simulink model "RBCM_Model"  (R2024b)
settings: Solver=FixedStepAuto  StartTime=0.0  StopTime=10.0  RelTol=1e-3
PreLoadFcn:
  | % NXP_MBDT_S32K3 callback: DO NOT REMOVE
  | mbd_s32k3.common.nxp.model_callbacks.preLoadFcn();
PostLoadFcn:
  | % NXP_MBDT_S32K3 callback: DO NOT REMOVE
  | mbd_s32k3.common.nxp.model_callbacks.postLoadFcn();
InitFcn:
  | % NXP_MBDT_S32K3 callback: DO NOT REMOVE
  | mbd_s32k3.common.nxp.model_callbacks.initFcn();
undefined symbols (not defined in the file or in its folder): AccuFanPwr_hHsd3ch2, BspdPwr_lHsd1ch2, BuzzerPwr_lHsd3ch3, DevicePwr_12v_lHsd1ch1, DevicePwr_hHsd1ch2, DrsPwr_8v_lHsd3ch1, hHsd_Diagnose_AdcBuffer, ILPwr_hHsd1ch1, lHsd_Diagnose_AdcBuffer, LoggerPwr_lHsd1ch3, PumpFan1_hHsd4ch1, PumpFan2_hHsd4ch2, PumpPwr_hHsd3ch1, RGBLED0state, TaillightPwr_lHsd3ch4, TempSensorPwr_lHsd1ch4
libraries: mbd_s32k3_io_library x127, simulink x48, canmsglib x8, mbd_s32k3_communication_library x7, mbd_s32k3_isr_library x6, mbd_s32k3_cdd_library x3, mbd_s32k3_utility_library x1
(part 2 of 10)

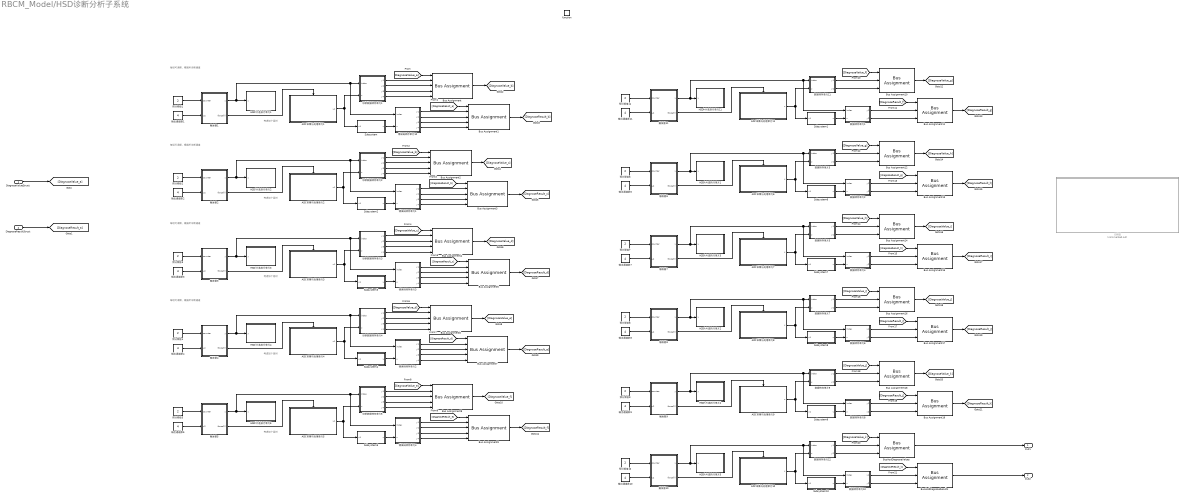
== system RBCM_Model/HSD诊断分析子系统 ==
  note: 考虑加个延时
  note: 每组可调频，根据所诊断通道
  note: 考虑加个延时
  note: 每组可调频，根据所诊断通道
  note: 考虑加个延时
  note: 每组可调频，根据所诊断通道
  note: 考虑加个延时
  note: 每组可调频，根据所诊断通道
  note: 考虑加个延时
  DiagnoseValueStruct : Inport  OutDataTypeStr=Bus: Bus_Hsd_Diagnose_Values
  DiagnoseResultStruct : Inport  Port=2  OutDataTypeStr=Bus: Bus_Hsd_Diagnose_Results
  function : TriggerPort  TriggerType=function-call  VariantControl=Variant
  ADC采集与处理单元1 : Subsystem
  ADC采集与处理单元10 : Subsystem
  ADC采集与处理单元11 : Subsystem
  ADC采集与处理单元2 : Subsystem
  ADC采集与处理单元3 : Subsystem
  ADC采集与处理单元4 : Subsystem
  ADC采集与处理单元5 : Subsystem
  ADC采集与处理单元6 : Subsystem
  ADC采集与处理单元7 : Subsystem
  ADC采集与处理单元8 : Subsystem
  ADC采集与处理单元9 : Subsystem
  Bus Assignment{,1..9} (10 alike) : BusAssignment  AssignedSignals=DevicePwr_12v_lHsd1ch1,BspdPwr_lHsd1ch2,LoggerPwr_lHsd1ch3,TempSensorPwr_lHsd1ch4
  Bus Assignment{10..19} (10 alike) : BusAssignment  AssignedSignals=ILPwr_hHsd1ch1,DevicePwr_hHsd1ch2
  BusHsdDiagnoseResults : BusAssignment  AssignedSignals=ILPwr_hHsd1ch1,DevicePwr_hHsd1ch2
  BusHsdDiagnoseValues : BusAssignment  AssignedSignals=ILPwr_hHsd1ch1,DevicePwr_hHsd1ch2
  HSDh片选执行单元1 : Subsystem
  HSDh片选执行单元11 : Subsystem
  HSDh片选执行单元2 : Subsystem
  HSDh片选执行单元3 : Subsystem
  HSDh片选执行单元4 : Subsystem
  HSDh片选执行单元5 : Subsystem
  HSDl片选执行单元1 : Subsystem
  HSDl片选执行单元2 : Subsystem
  HSDl片选执行单元3 : Subsystem
  HSDl片选执行单元4 : Subsystem
  HSDl片选执行单元5 : Subsystem
  Subsystem : Subsystem
  Subsystem1 : Subsystem
  Subsystem10 : Subsystem
  Subsystem2 : Subsystem
  Subsystem3 : Subsystem
  Subsystem4 : Subsystem
  Subsystem5 : Subsystem
  Subsystem6 : Subsystem
  Subsystem7 : Subsystem
  Subsystem8 : Subsystem
  Subsystem9 : Subsystem
  数据转存单元1 : MATLAB Function  TreatAsAtomicUnit=on
  数据转存单元10 : MATLAB Function  TreatAsAtomicUnit=on
  数据转存单元11 : MATLAB Function  TreatAsAtomicUnit=on
  数据转存单元12 : MATLAB Function  TreatAsAtomicUnit=on
  数据转存单元2 : MATLAB Function  TreatAsAtomicUnit=on
  数据转存单元3 : MATLAB Function  TreatAsAtomicUnit=on
  数据转存单元4 : MATLAB Function  TreatAsAtomicUnit=on
  数据转存单元5 : MATLAB Function  TreatAsAtomicUnit=on
  数据转存单元6 : MATLAB Function  TreatAsAtomicUnit=on
  数据转存单元7 : MATLAB Function  TreatAsAtomicUnit=on
  数据转存单元8 : MATLAB Function  TreatAsAtomicUnit=on
  数据转存单元9 : MATLAB Function  TreatAsAtomicUnit=on
  旧模型 : Subsystem  Commented=on
  触发器1 : MATLAB Function  TreatAsAtomicUnit=on
  触发器10 : MATLAB Function  TreatAsAtomicUnit=on
  触发器11 : MATLAB Function  TreatAsAtomicUnit=on
  触发器2 : MATLAB Function  TreatAsAtomicUnit=on
  触发器3 : MATLAB Function  TreatAsAtomicUnit=on
  触发器4 : MATLAB Function  TreatAsAtomicUnit=on
  触发器5 : MATLAB Function  TreatAsAtomicUnit=on
  触发器6 : MATLAB Function  TreatAsAtomicUnit=on
  触发器7 : MATLAB Function  TreatAsAtomicUnit=on
  触发器8 : MATLAB Function  TreatAsAtomicUnit=on
  触发器9 : MATLAB Function  TreatAsAtomicUnit=on
  诊断数据转存单元1 : MATLAB Function  TreatAsAtomicUnit=on
  诊断数据转存单元2 : MATLAB Function  TreatAsAtomicUnit=on
  诊断数据转存单元3 : MATLAB Function  TreatAsAtomicUnit=on
  诊断数据转存单元4 : MATLAB Function  TreatAsAtomicUnit=on
  诊断数据转存单元5 : MATLAB Function  TreatAsAtomicUnit=on
  输出通道数{1..11} (11 alike) : Constant  Value=4  OutDataTypeStr=uint8
  错误码转存单元1 : MATLAB Function  TreatAsAtomicUnit=on
  错误码转存单元10 : MATLAB Function  TreatAsAtomicUnit=on
  错误码转存单元2 : MATLAB Function  TreatAsAtomicUnit=on
  错误码转存单元3 : MATLAB Function  TreatAsAtomicUnit=on
  错误码转存单元4 : MATLAB Function  TreatAsAtomicUnit=on
  预分频值{1..11} (11 alike) : Constant  Value=2  OutDataTypeStr=uint8
  Out1 : Outport
  Out2 : Outport  Port=2
  wires:
  触发器1/2(fcncall()) -> ADC采集与处理单元1/Trigger
  触发器11/2(fcncall()) -> ADC采集与处理单元11/Trigger
  触发器11/1(y) -> HSDh片选执行单元11/1(y), 数据转存单元1/1(index), 数据转存单元11/1(index)
  触发器1/1(y) -> HSDl片选执行单元1/1(y), 错误码转存单元10/1(index), 诊断数据转存单元1/1(index)
  预分频值1/1 -> 触发器1/1(counter)
  预分频值11/1 -> 触发器11/1(counter)
  输出通道数11/1 -> 触发器11/2(u2)
  输出通道数1/1 -> 触发器1/2(u2)
  数据转存单元11/2(y2) -> Bus Assignment10/3
  数据转存单元11/1(y1) -> Bus Assignment10/2
  ADC采集与处理单元1/1(u1) -> 诊断数据转存单元1/2(u), Subsystem/1(u1)
  ADC采集与处理单元11/1(u) -> Subsystem1/1(u1), 数据转存单元11/2(u)
  Subsystem/1(u) -> 错误码转存单元10/2(u)
  Subsystem1/1(u) -> 数据转存单元1/2(u)
  数据转存单元1/1(y1) -> Bus Assignment11/2
  数据转存单元1/2(y2) -> Bus Assignment11/3
  错误码转存单元10/1(y1) -> Bus Assignment1/2
  诊断数据转存单元1/1(y1) -> Bus Assignment/2
  诊断数据转存单元1/2(y2) -> Bus Assignment/3
  诊断数据转存单元1/3(y3) -> Bus Assignment/4
  诊断数据转存单元1/4(y4) -> Bus Assignment/5
  Subsystem2/1(u) -> 错误码转存单元1/2(u)
  输出通道数2/1 -> 触发器2/2(u2)
  预分频值2/1 -> 触发器2/1(counter)
  触发器2/1(y) -> 诊断数据转存单元2/1(index), 错误码转存单元1/1(index), HSDl片选执行单元2/1(y)
  触发器2/2(fcncall()) -> ADC采集与处理单元2/Trigger
  触发器4/2(fcncall()) -> ADC采集与处理单元4/Trigger
  触发器4/1(y) -> HSDl片选执行单元4/1(y), 诊断数据转存单元4/1(index), 错误码转存单元2/1(index)
  预分频值4/1 -> 触发器4/1(counter)
  输出通道数4/1 -> 触发器4/2(u2)
  ADC采集与处理单元4/1(u1) -> 诊断数据转存单元4/2(u), Subsystem4/1(u1)
  Subsystem4/1(u) -> 错误码转存单元2/2(u)
  Subsystem3/1(u) -> 错误码转存单元3/2(u)
  ADC采集与处理单元3/1(u1) -> 诊断数据转存单元3/2(u), Subsystem3/1(u1)
  输出通道数3/1 -> 触发器3/2(u2)
  预分频值3/1 -> 触发器3/1(counter)
  触发器3/1(y) -> 诊断数据转存单元3/1(index), 错误码转存单元3/1(index), HSDl片选执行单元3/1(y)
  触发器3/2(fcncall()) -> ADC采集与处理单元3/Trigger
  Subsystem5/1(u) -> 错误码转存单元4/2(u)
  输出通道数5/1 -> 触发器5/2(u2)
  预分频值5/1 -> 触发器5/1(counter)
  触发器5/1(y) -> 诊断数据转存单元5/1(index), 错误码转存单元4/1(index), HSDl片选执行单元5/1(y)
  触发器5/2(fcncall()) -> ADC采集与处理单元5/Trigger
  Subsystem6/1(u) -> 数据转存单元2/2(u)
  ADC采集与处理单元6/1(u) -> 数据转存单元3/2(u), Subsystem6/1(u1)
  输出通道数6/1 -> 触发器6/2(u2)
  预分频值6/1 -> 触发器6/1(counter)
  触发器6/1(y) -> 数据转存单元3/1(index), 数据转存单元2/1(index), HSDh片选执行单元1/1(y)
  触发器6/2(fcncall()) -> ADC采集与处理单元6/Trigger
  触发器8/2(fcncall()) -> ADC采集与处理单元8/Trigger
  触发器8/1(y) -> HSDh片选执行单元2/1(y), 数据转存单元6/1(index), 数据转存单元7/1(index)
  预分频值8/1 -> 触发器8/1(counter)
  输出通道数8/1 -> 触发器8/2(u2)
  ADC采集与处理单元8/1(u) -> Subsystem8/1(u1), 数据转存单元7/2(u)
  Subsystem8/1(u) -> 数据转存单元6/2(u)
  Subsystem7/1(u) -> 数据转存单元4/2(u)
  ADC采集与处理单元7/1(u) -> 数据转存单元5/2(u), Subsystem7/1(u1)
  输出通道数7/1 -> 触发器7/2(u2)
  预分频值7/1 -> 触发器7/1(counter)
  触发器7/1(y) -> 数据转存单元5/1(index), 数据转存单元4/1(index), HSDh片选执行单元3/1(y)
  触发器7/2(fcncall()) -> ADC采集与处理单元7/Trigger
  Subsystem9/1(u) -> 数据转存单元8/2(u)
  ADC采集与处理单元9/1(u) -> 数据转存单元9/2(u), Subsystem9/1(u1)
  输出通道数9/1 -> 触发器9/2(u2)
  预分频值9/1 -> 触发器9/1(counter)
  触发器9/1(y) -> 数据转存单元9/1(index), 数据转存单元8/1(index), HSDh片选执行单元4/1(y)
  触发器9/2(fcncall()) -> ADC采集与处理单元9/Trigger
  触发器10/2(fcncall()) -> ADC采集与处理单元10/Trigger
  触发器10/1(y) -> HSDh片选执行单元5/1(y), 数据转存单元10/1(index), 数据转存单元12/1(index)
  预分频值10/1 -> 触发器10/1(counter)
  输出通道数10/1 -> 触发器10/2(u2)
  ADC采集与处理单元10/1(u) -> Subsystem10/1(u1), 数据转存单元12/2(u)
  Subsystem10/1(u) -> 数据转存单元10/2(u)
  DiagnoseValueStruct/1 -> [DiagnoseValue_a]
  DiagnoseResultStruct/1 -> [DiagnoseResult_a]
  [DiagnoseValue_a] -> Bus Assignment/1
  [DiagnoseResult_a] -> Bus Assignment1/1
  错误码转存单元10/2(y2) -> Bus Assignment1/3
  错误码转存单元10/3(y3) -> Bus Assignment1/4
  错误码转存单元10/4(y4) -> Bus Assignment1/5
  诊断数据转存单元2/2(y2) -> Bus Assignment2/3
  [DiagnoseResult_b] -> Bus Assignment3/1
  诊断数据转存单元2/1(y1) -> Bus Assignment2/2
  诊断数据转存单元2/4(y4) -> Bus Assignment2/5
  诊断数据转存单元2/3(y3) -> Bus Assignment2/4
  错误码转存单元1/4(y4) -> Bus Assignment3/5
  错误码转存单元1/2(y2) -> Bus Assignment3/3
  错误码转存单元1/1(y1) -> Bus Assignment3/2
  错误码转存单元1/3(y3) -> Bus Assignment3/4
  [DiagnoseValue_b] -> Bus Assignment2/1
  诊断数据转存单元3/2(y2) -> Bus Assignment4/3
  [DiagnoseResult_c] -> Bus Assignment5/1
  诊断数据转存单元3/1(y1) -> Bus Assignment4/2
  诊断数据转存单元3/4(y4) -> Bus Assignment4/5
  诊断数据转存单元3/3(y3) -> Bus Assignment4/4
  错误码转存单元3/4(y4) -> Bus Assignment5/5
  错误码转存单元3/2(y2) -> Bus Assignment5/3
  错误码转存单元3/1(y1) -> Bus Assignment5/2
  错误码转存单元3/3(y3) -> Bus Assignment5/4
  [DiagnoseValue_c] -> Bus Assignment4/1
  诊断数据转存单元4/2(y2) -> Bus Assignment6/3
  [DiagnoseResult_d] -> Bus Assignment7/1
  诊断数据转存单元4/1(y1) -> Bus Assignment6/2
  诊断数据转存单元4/4(y4) -> Bus Assignment6/5
  诊断数据转存单元4/3(y3) -> Bus Assignment6/4
  错误码转存单元2/4(y4) -> Bus Assignment7/5
  错误码转存单元2/2(y2) -> Bus Assignment7/3
  错误码转存单元2/1(y1) -> Bus Assignment7/2
  错误码转存单元2/3(y3) -> Bus Assignment7/4
  [DiagnoseValue_d] -> Bus Assignment6/1
  诊断数据转存单元5/2(y2) -> Bus Assignment8/3
  [DiagnoseResult_e] -> Bus Assignment9/1
  诊断数据转存单元5/1(y1) -> Bus Assignment8/2
  诊断数据转存单元5/4(y4) -> Bus Assignment8/5
  诊断数据转存单元5/3(y3) -> Bus Assignment8/4
  错误码转存单元4/4(y4) -> Bus Assignment9/5
  错误码转存单元4/2(y2) -> Bus Assignment9/3
  错误码转存单元4/1(y1) -> Bus Assignment9/2
  错误码转存单元4/3(y3) -> Bus Assignment9/4
  [DiagnoseValue_e] -> Bus Assignment8/1
  Bus Assignment/1 -> [DiagnoseValue_b]
  Bus Assignment1/1 -> [DiagnoseResult_b]
  Bus Assignment2/1 -> [DiagnoseValue_c]
  Bus Assignment3/1 -> [DiagnoseResult_c]
  Bus Assignment4/1 -> [DiagnoseValue_d]
  Bus Assignment5/1 -> [DiagnoseResult_d]
  Bus Assignment6/1 -> [DiagnoseValue_e]
  Bus Assignment7/1 -> [DiagnoseResult_e]
  Bus Assignment8/1 -> [DiagnoseValue_f]
  Bus Assignment9/1 -> [DiagnoseResult_f]
  [DiagnoseValue_f] -> Bus Assignment10/1
  [DiagnoseResult_f] -> Bus Assignment11/1
  Bus Assignment10/1 -> [DiagnoseValue_g]
  Bus Assignment11/1 -> [DiagnoseResult_g]
  数据转存单元2/1(y1) -> Bus Assignment13/2
  数据转存单元2/2(y2) -> Bus Assignment13/3
  数据转存单元3/2(y2) -> Bus Assignment12/3
  Bus Assignment12/1 -> [DiagnoseValue_h]
  [DiagnoseValue_g] -> Bus Assignment12/1
  [DiagnoseResult_g] -> Bus Assignment13/1
  数据转存单元3/1(y1) -> Bus Assignment12/2
  Bus Assignment13/1 -> [DiagnoseResult_h]
  数据转存单元4/1(y1) -> Bus Assignment15/2
  数据转存单元4/2(y2) -> Bus Assignment15/3
  数据转存单元5/2(y2) -> Bus Assignment14/3
  Bus Assignment14/1 -> [DiagnoseValue_i]
  [DiagnoseValue_h] -> Bus Assignment14/1
  [DiagnoseResult_h] -> Bus Assignment15/1
  数据转存单元5/1(y1) -> Bus Assignment14/2
  Bus Assignment15/1 -> [DiagnoseResult_i]
  数据转存单元6/1(y1) -> Bus Assignment17/2
  数据转存单元6/2(y2) -> Bus Assignment17/3
  数据转存单元7/2(y2) -> Bus Assignment16/3
  Bus Assignment16/1 -> [DiagnoseValue_j]
  [DiagnoseValue_i] -> Bus Assignment16/1
  [DiagnoseResult_i] -> Bus Assignment17/1
  数据转存单元7/1(y1) -> Bus Assignment16/2
  Bus Assignment17/1 -> [DiagnoseResult_j]
  数据转存单元8/1(y1) -> Bus Assignment19/2
  数据转存单元8/2(y2) -> Bus Assignment19/3
  数据转存单元9/2(y2) -> Bus Assignment18/3
  Bus Assignment18/1 -> [DiagnoseValue_k]
  [DiagnoseValue_j] -> Bus Assignment18/1
  [DiagnoseResult_j] -> Bus Assignment19/1
  数据转存单元9/1(y1) -> Bus Assignment18/2
  Bus Assignment19/1 -> [DiagnoseResult_k]
  数据转存单元10/1(y1) -> BusHsdDiagnoseResults/2
  数据转存单元10/2(y2) -> BusHsdDiagnoseResults/3
  数据转存单元12/2(y2) -> BusHsdDiagnoseValues/3
  BusHsdDiagnoseValues/1 -> Out1/1
  [DiagnoseValue_k] -> BusHsdDiagnoseValues/1
  [DiagnoseResult_k] -> BusHsdDiagnoseResults/1
  数据转存单元12/1(y1) -> BusHsdDiagnoseValues/2
  BusHsdDiagnoseResults/1 -> Out2/1
  ADC采集与处理单元2/1(u1) -> 诊断数据转存单元2/2(u), Subsystem2/1(u1)
  ADC采集与处理单元5/1(u1) -> 诊断数据转存单元5/2(u), Subsystem5/1(u1)

== system RBCM_Model/HSD诊断数据抓取与发送(不启用) ==
  Trigger : TriggerPort  TriggerType=function-call  VariantControl=(inherit)  PortDimensions=1
  Bus Selector : BusSelector  OutputSignals=Data,Length,ID
  CAN Pack2 : canmsglib/CAN Pack  CANdbFile=E:\Workspace\Myworkspace\RBCM_S32K344_AUTOSAR_MBD\Firmware\AUTOSAR_MBD\RBCM_ModelConfig\E10_dbc_240819_CAN.dbc  MsgList=BHVB_State  MsgName=BHVB_State  MsgIDType=Extended (29-bit identifier)  MsgIdentifier=536870911  CANIDInput=off  MsgLength=8  Remote=off  ApplyMinMax=off  BusOutput=on  SignalInfo={'HSDx_Channelx_State1','8','8','LE','unsigned','Standard','0','1','0','-Inf','Inf';'HSDx_Channelx_State2','16','8','LE','unsigned','Standard','0','1','0','-Inf','Inf';'HSDx_Channelx_State3','24','8','LE','unsigned','Standard','0','1','0','-Inf','Inf';'HSDx_Channelx_State4','32','8','LE','unsigned','Standard','0','1','0','-Inf','Inf';'HSDx_Channelx_State5','40','8','LE','unsigned','Standard','0','1','0','-Inf','Inf';'HSDx_Channelx_State6','48','8','LE','unsigned','Standard','0','1','0','-Inf','Inf';'PDB_State_Pack_number','0','8','LE','unsigned','Standard','0','1','0','0','255'}
      settings: LibrarySourceBlock=canlib/CAN Pack  DataFormat=CANdb specified signals
  Can : mbd_s32k3_communication_library/Can  api_func=Can_Write  controller=No controller configured  hw_obj=CanHardwareObject_Can0_Tx_Interrupt  mode=CAN_CS_STARTED  canfd_msg=off  ext_id_msg=off  empty_msg=off  text=|
      | CanConfigSet - CanConfigSet 
      | CanConfigSet/CanController - CanController_0 
      | CanConfigSet/CanController_0/CanAutoBusOffRecovery - false 
      | CanConfigSet/CanController_0/CanBusoffProcessing - POLLING 
      | CanConfigSet/CanController_0/CanControllerActivation - true 
      | CanConfigSet/CanController_0/CanControllerBaseAddress - 0 
      | CanConfigSet/CanController_0/CanControllerBaudrateConfig - CanControllerBaudrateConfig_0 
      | CanConfigSet/CanController_0/CanControllerBaudrateConfig_0/CanAdvancedSetting - false 
      | CanConfigSet/CanController_0/CanControllerBaudrateConfig_0/CanBaudrateTypeSuport - NORMAL_CBT 
      | CanConfigSet/CanController_0/CanControllerBaudrateConfig_0/CanBusLength - 40 
      | CanConfigSet/CanController_0/CanControllerBaudrateConfig_0/CanControllerBaudRate - 500.0 
      | CanConfigSet/CanController_0/CanControllerBaudrateConfig_0/CanControllerBaudRateConfigID - 0 
      | CanConfigSet/CanController_0/CanControllerBaudrateConfig_0/CanControllerFdBaudrateConfig - CanControllerFdBaudrateConfig 
      | CanConfigSet/CanController_0/CanControllerBaudrateConfig_0/CanControllerFdBaudrateConfig/CanControllerFdBaudRate - 2000 
      | CanConfigSet/CanController_0/CanControllerBaudrateConfig_0/CanControllerFdBaudrateConfig/CanControllerFdPrescaller - 2 
      | CanConfigSet/CanController_0/CanControllerBaudrateConfig_0/CanControllerFdBaudrateConfig/CanControllerFdSyncSeg - 1 
      | CanConfigSet/CanController_0/CanControllerBaudrateConfig_0/CanControllerFdBaudrateConfig/CanControllerPrescallerAlternateFd - 1 
      | CanConfigSet/CanController_0/CanControllerBaudrateConfig_0/CanControllerFdBaudrateConfig/CanControllerPropSeg - 5 
      | CanConfigSet/CanController_0/CanControllerBaudrateConfig_0/CanControllerFdBaudrateConfig/CanControllerSeg1 - 2 
      | CanConfigSet/CanController_0/CanControllerBaudrateConfig_0/CanControllerFdBaudrateConfig/CanControllerSeg2 - 2 
      | CanConfigSet/CanController_0/CanControllerBaudrateConfig_0/CanControllerFdBaudrateConfig/CanControllerSyncJumpWidth - 2 
      | CanConfigSet/CanController_0/CanControllerBaudrateConfig_0/CanControllerFdBaudrateConfig/CanControllerTxBitRateSwitch - true 
      | CanConfigSet/CanController_0/CanControllerBaudrateConfig_0/CanControllerFdBaudrateConfig/Index - 0 
      | CanConfigSet/CanController_0/CanControllerBaudrateConfig_0/CanControllerPrescaller - 2 
      | CanConfigSet/CanController_0/CanControllerBaudrateConfig_0/CanControllerPrescallerAlternate - 10 
      | CanConfigSet/CanController_0/CanControllerBaudrateConfig_0/CanControllerPropSeg - 11 
      | CanConfigSet/CanController_0/CanControllerBaudrateConfig_0/CanControllerSeg1 - 18 
      | CanConfigSet/CanController_0/CanControllerBaudrateConfig_0/CanControllerSeg2 - 10 
      | CanConfigSet/CanController_0/CanControllerBaudrateConfig_0/CanControllerSyncJumpWidth - 10 
      | CanConfigSet/CanController_0/CanControllerBaudrateConfig_0/CanControllerSyncSeg - 1 
      | CanConfigSet/CanController_0/CanControllerBaudrateConfig_0/CanPropDelayTranceiver - 150.0 
      | CanConfigSet/CanController_0/CanControllerBaudrateConfig_0/CanTxArbitrationStartDelay - 12 
      | CanConfigSet/CanController_0/CanControllerBaudrateConfig_0/Index - 0 
      | CanConfigSet/CanController_0/CanControllerDefaultBaudrate - /Can_43_FLEXCAN/Can/CanConfigSet/CanController_0/CanControllerBaudrateConfig_0 
      | CanConfigSet/CanController_0/CanControllerEdgeFilter - false 
      | CanConfigSet/CanController_0/CanControllerFdISO - true 
      | CanConfigSet/CanController_0/CanControllerId - 0 
      | CanConfigSet/CanController_0/CanControllerPrExcEn - false 
      | CanConfigSet/CanController_0/CanCpuClockRef - /Mcu/Mcu/McuModuleConfiguration/McuClockSettingConfig_0/FLEXCAN_PE_CLK0_2 
      | CanConfigSet/CanController_0/CanCpuClockRefAlternate - /Mcu/Mcu/McuModuleConfiguration/McuClockSettingConfig_0/FLEXCAN_PE_CLK0_2 
      | CanConfigSet/CanController_0/CanHwChannel - FLEXCAN_0 
      | CanConfigSet/CanController_0/CanLoopBackMode - false 
      | CanConfigSet/CanController_0/CanRamBlock - CanRamBlock 
      | CanConfigSet/CanController_0/CanRamBlock/CanRamBlockUnified - CanRamBlockUnified 
      | CanConfigSet/CanController_0/CanRamBlock/CanRamBlockUnified/CanBlockUnifiedPayloadLength - CAN_16_BYTES_PAYLOAD 
      | CanConfigSet/CanController_0/CanRamBlock/Choice - CanRamBlockUnified 
      | CanConfigSet/CanController_0/CanRamBlock/Index - 0 
      | CanConfigSet/CanController_0/CanRxFiFo - CanRxFiFo 
      | CanConfigSet/CanController_0/CanRxFiFo/CanEnhanceFiFo - CanRxFiFo 
      | CanConfigSet/CanController_0/CanRxFiFo/CanRxFiFo/CanEnhanceFiFoDmaEnable - false 
      | CanConfigSet/CanController_0/CanRxFiFo/CanRxFiFo/CanEnhancedSchemeType - MASK_FILTER_SCHEME 
      | CanConfigSet/CanController_0/CanRxFiFo/CanRxFiFo/CanFiFoDmaErrorNotif - NULL_PTR 
      | CanConfigSet/CanController_0/CanRxFiFo/CanRxFiFo/CanFiFoOverflowNotif - MBDT_FlexCAN0_FifoOverflowNotif 
      | CanConfigSet/CanController_0/CanRxFiFo/CanRxFiFo/NumberMBTransferDMA - 1 
      | CanConfigSet/CanController_0/CanRxFiFo/Choice - CanEnhanceFiFo 
      | CanConfigSet/CanController_0/CanRxFiFo/Index - 0 
      | CanConfigSet/CanController_0/CanRxProcessing - MIXED 
      | CanConfigSet/CanController_0/CanTrippleSamplingEnable - false 
      | CanConfigSet/CanController_0/CanTxProcessing - MIXED 
      | CanConfigSet/CanController_0/CanWakeupFunctionalityAPI - false 
      | CanConfigSet/CanController_0/CanWakeupProcessing - POLLING 
      | CanConfigSet/CanController_0/CanWakeupSupport - false 
      | CanConfigSet/CanController_0/Index - 0 
      | CanConfigSet/CanHardwareObject - CanHardwareObject_Can0_Rx_Ext_Interrupt CanHardwareObject_Can0_Rx_FIFO CanHardwareObject_Can0_Rx_Std_Polling CanHardwareObject_Can0_Tx_Interrupt CanHardwareObject_Can0_Tx_Polling 
      | CanConfigSet/CanHardwareObject_Can0_Rx_Ext_Interrupt/CanControllerRef - /Can_43_FLEXCAN/Can/CanConfigSet/CanController_0 
      | CanConfigSet/CanHardwareObject_Can0_Rx_Ext_Interrupt/CanHandleType - BASIC 
      | CanConfigSet/CanHardwareObject_Can0_Rx_Ext_Interrupt/CanHardwareObjectUsesPolling - false 
      | CanConfigSet/CanHardwareObject_Can0_Rx_Ext_Interrupt/CanHwFilter - CanHwFilter_0 
      | CanConfigSet/CanHardwareObject_Can0_Rx_Ext_Interrupt/CanHwFilter_0/CanHwFilterCode - 0 
      | CanConfigSet/CanHardwareObject_Can0_Rx_Ext_Interrupt/CanHwFilter_0/CanHwFilterMask - 0 
      | CanConfigSet/CanHardwareObject_Can0_Rx_Ext_Interrupt/CanHwFilter_0/Index - 0 
      | CanConfigSet/CanHardwareObject_Can0_Rx_Ext_Interrupt/CanHwObjectCount - 1 
      | CanConfigSet/CanHardwareObject_Can0_Rx_Ext_Interrupt/CanIdType - EXTENDED 
      | CanConfigSet/CanHardwareObject_Can0_Rx_Ext_Interrupt/CanObjectId - 2 
      | CanConfigSet/CanHardwareObject_Can0_Rx_Ext_Interrupt/CanObjectType - RECEIVE 
      | CanConfigSet/CanHardwareObject_Can0_Rx_Ext_Interrupt/Index - 2 
      | CanConfigSet/CanHardwareObject_Can0_Rx_FIFO/CanControllerRef - /Can_43_FLEXCAN/Can/CanConfigSet/CanController_0 
      | CanConfigSet/CanHardwareObject_Can0_Rx_FIFO/CanHandleType - BASIC 
      | CanConfigSet/CanHardwareObject_Can0_Rx_FIFO/CanHardwareObjectUsesPolling - false 
      | CanConfigSet/CanHardwareObject_Can0_Rx_FIFO/CanHwFilter - CanHwFilter_0 CanHwFilter_1 CanHwFilter_2 CanHwFilter_3 CanHwFilter_4 CanHwFilter_5 CanHwFilter_6 CanHwFilter_7 
      | CanConfigSet/CanHardwareObject_Can0_Rx_FIFO/CanHwFilter_0/CanHwFilterCode - 1008 
      | CanConfigSet/CanHardwareObject_Can0_Rx_FIFO/CanHwFilter_0/CanHwFilterMask - 536870911 
      | CanConfigSet/CanHardwareObject_Can0_Rx_FIFO/CanHwFilter_0/Index - 0 
      | CanConfigSet/CanHardwareObject_Can0_Rx_FIFO/CanHwFilter_1/CanHwFilterCode - 1009 
      | CanConfigSet/CanHardwareObject_Can0_Rx_FIFO/CanHwFilter_1/CanHwFilterMask - 536870911 
      | CanConfigSet/CanHardwareObject_Can0_Rx_FIFO/CanHwFilter_1/Index - 1 
      | CanConfigSet/CanHardwareObject_Can0_Rx_FIFO/CanHwFilter_2/CanHwFilterCode - 1010 
      | CanConfigSet/CanHardwareObject_Can0_Rx_FIFO/CanHwFilter_2/CanHwFilterMask - 536870911 
      | CanConfigSet/CanHardwareObject_Can0_Rx_FIFO/CanHwFilter_2/Index - 2 
      | CanConfigSet/CanHardwareObject_Can0_Rx_FIFO/CanHwFilter_3/CanHwFilterCode - 1011 
      | CanConfigSet/CanHardwareObject_Can0_Rx_FIFO/CanHwFilter_3/CanHwFilterMask - 536870911 
      | CanConfigSet/CanHardwareObject_Can0_Rx_FIFO/CanHwFilter_3/Index - 3 
      | CanConfigSet/CanHardwareObject_Can0_Rx_FIFO/CanHwFilter_4/CanHwFilterCode - 1012 
      | CanConfigSet/CanHardwareObject_Can0_Rx_FIFO/CanHwFilter_4/CanHwFilterMask - 536870911 
      | CanConfigSet/CanHardwareObject_Can0_Rx_FIFO/CanHwFilter_4/Index - 4 
      | CanConfigSet/CanHardwareObject_Can0_Rx_FIFO/CanHwFilter_5/CanHwFilterCode - 1013 
      | CanConfigSet/CanHardwareObject_Can0_Rx_FIFO/CanHwFilter_5/CanHwFilterMask - 536870911 
      | CanConfigSet/CanHardwareObject_Can0_Rx_FIFO/CanHwFilter_5/Index - 5 
      | CanConfigSet/CanHardwareObject_Can0_Rx_FIFO/CanHwFilter_6/CanHwFilterCode - 1014 
      | CanConfigSet/CanHardwareObject_Can0_Rx_FIFO/CanHwFilter_6/CanHwFilterMask - 536870911 
      | CanConfigSet/CanHardwareObject_Can0_Rx_FIFO/CanHwFilter_6/Index - 6 
      | CanConfigSet/CanHardwareObject_Can0_Rx_FIFO/CanHwFilter_7/CanHwFilterCode - 1015 
      | CanConfigSet/CanHardwareObject_Can0_Rx_FIFO/CanHwFilter_7/CanHwFilterMask - 536870911 
      | CanConfigSet/CanHardwareObject_Can0_Rx_FIFO/CanHwFilter_7/Index - 7 
      | CanConfigSet/CanHardwareObject_Can0_Rx_FIFO/CanHwObjectCount - 6 
      | CanConfigSet/CanHardwareObject_Can0_Rx_FIFO/CanIdType - EXTENDED 
      | CanConfigSet/CanHardwareObject_Can0_Rx_FIFO/CanObjectId - 0 
      | CanConfigSet/CanHardwareObject_Can0_Rx_FIFO/CanObjectType - RECEIVE 
      | CanConfigSet/CanHardwareObject_Can0_Rx_FIFO/Index - 0 
      | CanConfigSet/CanHardwareObject_Can0_Rx_Std_Polling/CanControllerRef - /Can_43_FLEXCAN/Can/CanConfigSet/CanController_0 
      | CanConfigSet/CanHardwareObject_Can0_Rx_Std_Polling/CanHandleType - BASIC 
      | CanConfigSet/CanHardwareObject_Can0_Rx_Std_Polling/CanHardwareObjectUsesPolling - true 
      | CanConfigSet/CanHardwareObject_Can0_Rx_Std_Polling/CanHwFilter - CanHwFilter_0 
      | CanConfigSet/CanHardwareObject_Can0_Rx_Std_Polling/CanHwFilter_0/CanHwFilterCode - 0 
      | CanConfigSet/CanHardwareObject_Can0_Rx_Std_Polling/CanHwFilter_0/CanHwFilterMask - 0 
      | CanConfigSet/CanHardwareObject_Can0_Rx_Std_Polling/CanHwFilter_0/Index - 0 
      | CanConfigSet/CanHardwareObject_Can0_Rx_Std_Polling/CanHwObjectCount - 1 
      | CanConfigSet/CanHardwareObject_Can0_Rx_Std_Polling/CanIdType - STANDARD 
      | CanConfigSet/CanHardwareObject_Can0_Rx_Std_Polling/CanMainFunctionRWPeriodRef - /Can_43_FLEXCAN/Can/CanGeneral/CanMainFunctionRWPeriods_0 
      | CanConfigSet/CanHardwareObject_Can0_Rx_Std_Polling/CanObjectId - 1 
      | CanConfigSet/CanHardwareObject_Can0_Rx_Std_Polling/CanObjectType - RECEIVE 
      | CanConfigSet/CanHardwareObject_Can0_Rx_Std_Polling/Index - 1 
      | CanConfigSet/CanHardwareObject_Can0_Tx_Interrupt/CanControllerRef - /Can_43_FLEXCAN/Can/CanConfigSet/CanController_0 
      | CanConfigSet/CanHardwareObject_Can0_Tx_Interrupt/CanHandleType - BASIC 
      | CanConfigSet/CanHardwareObject_Can0_Tx_Interrupt/CanHardwareObjectUsesPolling - false 
      | CanConfigSet/CanHardwareObject_Can0_Tx_Interrupt/CanHwObjectCount - 1 
      | CanConfigSet/CanHardwareObject_Can0_Tx_Interrupt/CanIdType - MIXED 
      | CanConfigSet/CanHardwareObject_Can0_Tx_Interrupt/CanObjectId - 4 
      | CanConfigSet/CanHardwareObject_Can0_Tx_Interrupt/CanObjectType - TRANSMIT 
      | CanConfigSet/CanHardwareObject_Can0_Tx_Interrupt/Index - 4 
      | CanConfigSet/CanHardwareObject_Can0_Tx_Polling/CanControllerRef - /Can_43_FLEXCAN/Can/CanConfigSet/CanController_0 
      | CanConfigSet/CanHardwareObject_Can0_Tx_Polling/CanHandleType - BASIC 
      | CanConfigSet/CanHardwareObject_Can0_Tx_Polling/CanHardwareObjectUsesPolling - true 
      | CanConfigSet/CanHardwareObject_Can0_Tx_Polling/CanHwObjectCount - 1 
      | CanConfigSet/CanHardwareObject_Can0_Tx_Polling/CanIdType - MIXED 
      | CanConfigSet/CanHardwareObject_Can0_Tx_Polling/CanMainFunctionRWPeriodRef - /Can_43_FLEXCAN/Can/CanGeneral/CanMainFunctionRWPeriods_0 
      | CanConfigSet/CanHardwareObject_Can0_Tx_Polling/CanObjectId - 3 
      | CanConfigSet/CanHardwareObject_Can0_Tx_Polling/CanObjectType - TRANSMIT 
      | CanConfigSet/CanHardwareObject_Can0_Tx_Polling/Index - 3 
      | CanGeneral - CanGeneral 
      | CanGeneral/CanApiEnableMbAbort - true 
      | CanGeneral/CanDevErrorDetect - true 
      | CanGeneral/CanEnableDualClockMode - false 
      | CanGeneral/CanEnableSecurityEventReporting - false 
      | CanGeneral/CanEnableUserModeSupport - false 
      | CanGeneral/CanGlobalTimeSupport - false 
      | CanGeneral/CanIndex - 0 
      | CanGeneral/CanMBCountExtensionSupport - false 
      | CanGeneral/CanMainFunctionModePeriod - 0.001 
      | CanGeneral/CanMainFunctionRWPeriods - CanMainFunctionRWPeriods_0 
      | CanGeneral/CanMainFunctionRWPeriods_0/CanMainFunctionPeriod - 0.001 
      | CanGeneral/CanMainFunctionRWPeriods_0/Index - 0 
      | CanGeneral/CanMultiPartitionSupport - false 
      | CanGeneral/CanMultiplexedTransmission - true 
      | CanGeneral/CanSetBaudrateApi - true 
      | CanGeneral/CanTimeoutDuration - 1.0 
      | CanGeneral/CanTimeoutMethod - OSIF_COUNTER_DUMMY 
      | CanGeneral/CanVersionInfoApi - true 
      | CommonPublishedInformation - CommonPublishedInformation 
      | CommonPublishedInformation/ArReleaseMajorVersion - 4 
      | CommonPublishedInformation/ArReleaseMinorVersion - 7 
      | CommonPublishedInformation/ArReleaseRevisionVersion - 0 
      | CommonPublishedInformation/ModuleId - 80 
      | CommonPublishedInformation/SwMajorVersion - 3 
      | CommonPublishedInformation/SwMinorVersion - 0 
      | CommonPublishedInformation/SwPatchVersion - 0 
      | CommonPublishedInformation/VendorApiInfix - FLEXCAN 
      | CommonPublishedInformation/VendorId - 43 
      | IMPLEMENTATION-CONFIG-VARIANT - VARIANT-POST-BUILD 
      | POST_BUILD_VARIANT_USED - true
      settings: SourceProductName=Communication Blocks
  Data Store Read{,1..5} (6 alike) : DataStoreRead  DataStoreName=HSD_diagnostic_data  DataStoreElements=HSD_diagnostic_data  EnableIndexing=on  IndexOptions=Index vector (port)  Indices=1  OutputSizes=1
  Data Store Write1 : DataStoreWrite  DataStoreName=can_id  IndexOptions=Index vector (dialog)  Indices=1  OutputSizes=1
  HSD总组数 : Constant  Value=5
  HSD组轮询单元 : MATLAB Function  TreatAsAtomicUnit=on
  HSD诊断数据索引单元 : Subsystem
  Terminator : Terminator
  Terminator2 : Terminator
  wires:
  HSD总组数/1 -> HSD组轮询单元/1(u)
  Data Store Read/1 -> CAN Pack2/2
  Data Store Read1/1 -> CAN Pack2/3
  Data Store Read2/1 -> CAN Pack2/4
  Data Store Read3/1 -> CAN Pack2/5
  Data Store Read4/1 -> CAN Pack2/6
  Data Store Read5/1 -> CAN Pack2/7
  HSD诊断数据索引单元/1(Out1) -> Data Store Read/1
  HSD诊断数据索引单元/2(Out2) -> Data Store Read1/1
  HSD组轮询单元/1(y) -> CAN Pack2/1, HSD诊断数据索引单元/1(y)
  HSD组轮询单元/2(fcncall()) -> HSD诊断数据索引单元/Trigger
  HSD诊断数据索引单元/3(Out3) -> Data Store Read2/1
  HSD诊断数据索引单元/4(Out4) -> Data Store Read3/1
  HSD诊断数据索引单元/5(Out5) -> Data Store Read4/1
  HSD诊断数据索引单元/6(Out6) -> Data Store Read5/1
  Bus Selector/1 -> Can/3  "<Data>"
  Can/1 -> Terminator/1
  Bus Selector/3 -> Can/1, Data Store Write1/1  "<ID>"
  CAN Pack2/1 -> Bus Selector/1
  Bus Selector/2 -> Terminator2/1  "<Length>"

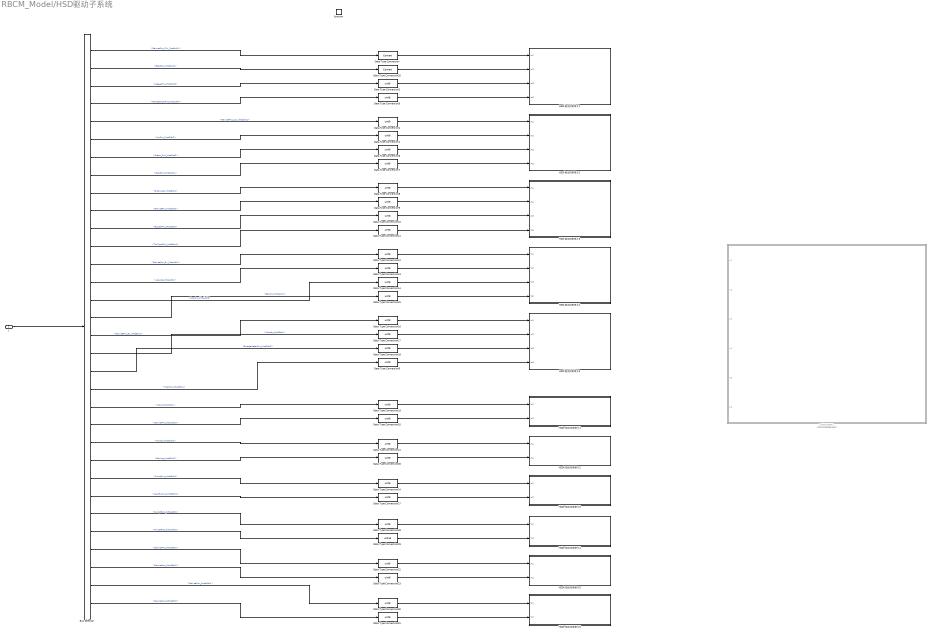
== system RBCM_Model/HSD驱动子系统 ==
  y : Inport  OutDataTypeStr=Bus: Bus_Hsd_Drive_Commands
  function : TriggerPort  TriggerType=function-call  VariantControl=Variant
  Bus Selector : BusSelector  OutputSignals=DevicePwr_12v_lHsd1ch1,BspdPwr_lHsd1ch2,LoggerPwr_lHsd1ch3,TempSensorPwr_lHsd1ch4,DevicePwr_12v_lHsd2ch1,VcuPwr_lHsd2ch2,Fireon_Pwr_lHsd2ch3,DsbdPwr_lHsd2ch4,DrsPwr_8v_lHsd3ch1,DevicePwr_lHsd3ch2,BuzzerPwr_lHsd3ch3,TaillightPwr_lHsd3ch4,DevicePwr_5v_lHsd4ch1,AccuUbr_lHsd4ch2,AccuPwr_lHsd4ch3,BduPwr_lHsd4ch4,DevicePwr_5v_lHsd5ch1,McuUbr_lHsd5ch2,EnergeMeterPwr_lHsd5ch3,TsalrPwr_lHsd5ch4,ILPwr_hHsd1ch1,DevicePwr_hHsd1ch2,VcuUbr_hHsd2ch1,Device_hHsd2ch2,PumpPwr_hHsd3ch1,AccuFanPwr_hHsd3ch2,PumpFan1_hHsd4ch1,PumpFan2_hHsd4ch2,DevicePwr_hHsd5ch1,DevicePwr_hHsd5ch2,DevicePwr_hHsd6ch1,DevicePwr_hHsd6ch2
  Data Type Conversion : DataTypeConversion  SaturateOnIntegerOverflow=off  RndMeth=Floor
  Data Type Conversion{1..24,26..28,30..31} (29 alike) : DataTypeConversion  OutDataTypeStr=uint8  SaturateOnIntegerOverflow=off  RndMeth=Floor
  Data Type Conversion25 : DataTypeConversion  SaturateOnIntegerOverflow=off  RndMeth=Floor
  Data Type Conversion29 : DataTypeConversion  OutDataTypeStr=uint16  SaturateOnIntegerOverflow=off  RndMeth=Floor
  HSDh输出控制单元1 : Subsystem
  HSDh输出控制单元2 : Subsystem
  HSDh输出控制单元3 : Subsystem
  HSDh输出控制单元4 : Subsystem
  HSDh输出控制单元5 : Subsystem
  HSDh输出控制单元6 : Subsystem
  HSDl输出控制单元1 : Subsystem
  HSDl输出控制单元2 : Subsystem
  HSDl输出控制单元3 : Subsystem
  HSDl输出控制单元4 : Subsystem
  HSDl输出控制单元5 : Subsystem
  Subsystem1 : Subsystem  Commented=on
  wires:
  Data Type Conversion18/1 -> HSDl输出控制单元5/3(In3)
  Data Type Conversion14/1 -> HSDl输出控制单元4/3(In3)
  Data Type Conversion11/1 -> HSDl输出控制单元3/4(In6)
  Data Type Conversion10/1 -> HSDl输出控制单元3/3(In3)
  Data Type Conversion24/1 -> HSDh输出控制单元3/1(In1)
  Data Type Conversion7/1 -> HSDl输出控制单元2/4(In6)
  Data Type Conversion26/1 -> HSDh输出控制单元2/2(In2)
  Data Type Conversion17/1 -> HSDl输出控制单元5/2(In2)
  Data Type Conversion19/1 -> HSDh输出控制单元1/1(In1)
  Data Type Conversion1/1 -> HSDl输出控制单元2/2(In2)
  Data Type Conversion/1 -> HSDl输出控制单元1/1(In1)
  Data Type Conversion16/1 -> HSDl输出控制单元5/1(In1)
  Data Type Conversion15/1 -> HSDl输出控制单元4/4(In6)
  Data Type Conversion27/1 -> HSDh输出控制单元3/2(In2)
  Data Type Conversion13/1 -> HSDl输出控制单元4/2(In2)
  Data Type Conversion22/1 -> HSDh输出控制单元5/1(In1)
  Data Type Conversion25/1 -> HSDl输出控制单元1/2(In2)
  Data Type Conversion5/1 -> HSDl输出控制单元5/4(In6)
  Data Type Conversion20/1 -> HSDh输出控制单元1/2(In2)
  Data Type Conversion4/1 -> HSDl输出控制单元2/1(In1)
  Data Type Conversion12/1 -> HSDl输出控制单元4/1(In1)
  Data Type Conversion21/1 -> HSDh输出控制单元2/1(In1)
  Data Type Conversion29/1 -> HSDh输出控制单元4/2(In2)
  Data Type Conversion6/1 -> HSDl输出控制单元2/3(In3)
  Data Type Conversion28/1 -> HSDh输出控制单元4/1(In1)
  Data Type Conversion3/1 -> HSDl输出控制单元1/4(In6)
  Data Type Conversion23/1 -> HSDh输出控制单元5/2(In2)
  Data Type Conversion8/1 -> HSDl输出控制单元3/1(In1)
  Data Type Conversion2/1 -> HSDl输出控制单元1/3(In3)
  y/1 -> Bus Selector/1
  Bus Selector/2 -> Data Type Conversion25/1  "<BspdPwr_lHsd1ch2>"
  Bus Selector/3 -> Data Type Conversion2/1  "<LoggerPwr_lHsd1ch3>"
  Bus Selector/4 -> Data Type Conversion3/1  "<TempSensorPwr_lHsd1ch4>"
  Bus Selector/5 -> Data Type Conversion4/1  "<DevicePwr_12v_lHsd2ch1>"
  Bus Selector/6 -> Data Type Conversion1/1  "<VcuPwr_lHsd2ch2>"
  Bus Selector/7 -> Data Type Conversion6/1  "<Fireon_Pwr_lHsd2ch3>"
  Bus Selector/8 -> Data Type Conversion7/1  "<DsbdPwr_lHsd2ch4>"
  Bus Selector/9 -> Data Type Conversion8/1  "<DrsPwr_8v_lHsd3ch1>"
  Data Type Conversion9/1 -> HSDl输出控制单元3/2(In2)
  Bus Selector/10 -> Data Type Conversion9/1  "<DevicePwr_lHsd3ch2>"
  Bus Selector/11 -> Data Type Conversion10/1  "<BuzzerPwr_lHsd3ch3>"
  Bus Selector/12 -> Data Type Conversion11/1  "<TaillightPwr_lHsd3ch4>"
  Bus Selector/13 -> Data Type Conversion12/1  "<DevicePwr_5v_lHsd4ch1>"
  Bus Selector/14 -> Data Type Conversion13/1  "<AccuUbr_lHsd4ch2>"
  Bus Selector/15 -> Data Type Conversion14/1  "<AccuPwr_lHsd4ch3>"
  Bus Selector/16 -> Data Type Conversion15/1  "<BduPwr_lHsd4ch4>"
  Bus Selector/17 -> Data Type Conversion16/1  "<DevicePwr_5v_lHsd5ch1>"
  Bus Selector/18 -> Data Type Conversion17/1  "<McuUbr_lHsd5ch2>"
  Bus Selector/19 -> Data Type Conversion18/1  "<EnergeMeterPwr_lHsd5ch3>"
  Bus Selector/20 -> Data Type Conversion5/1  "<TsalrPwr_lHsd5ch4>"
  Bus Selector/21 -> Data Type Conversion19/1  "<ILPwr_hHsd1ch1>"
  Bus Selector/22 -> Data Type Conversion20/1  "<DevicePwr_hHsd1ch2>"
  Bus Selector/23 -> Data Type Conversion21/1  "<VcuUbr_hHsd2ch1>"
  Bus Selector/24 -> Data Type Conversion26/1  "<Device_hHsd2ch2>"
  Bus Selector/25 -> Data Type Conversion24/1  "<PumpPwr_hHsd3ch1>"
  Bus Selector/26 -> Data Type Conversion27/1  "<AccuFanPwr_hHsd3ch2>"
  Bus Selector/27 -> Data Type Conversion28/1  "<PumpFan1_hHsd4ch1>"
  Bus Selector/28 -> Data Type Conversion29/1  "<PumpFan2_hHsd4ch2>"
  Bus Selector/29 -> Data Type Conversion22/1  "<DevicePwr_hHsd5ch1>"
  Bus Selector/30 -> Data Type Conversion23/1  "<DevicePwr_hHsd5ch2>"
  Bus Selector/1 -> Data Type Conversion/1  "<DevicePwr_12v_lHsd1ch1>"
  Bus Selector/32 -> Data Type Conversion31/1  "<DevicePwr_hHsd6ch2>"
  Data Type Conversion31/1 -> HSDh输出控制单元6/2(In2)
  Data Type Conversion30/1 -> HSDh输出控制单元6/1(In1)
  Bus Selector/31 -> Data Type Conversion30/1  "<DevicePwr_hHsd6ch1>"

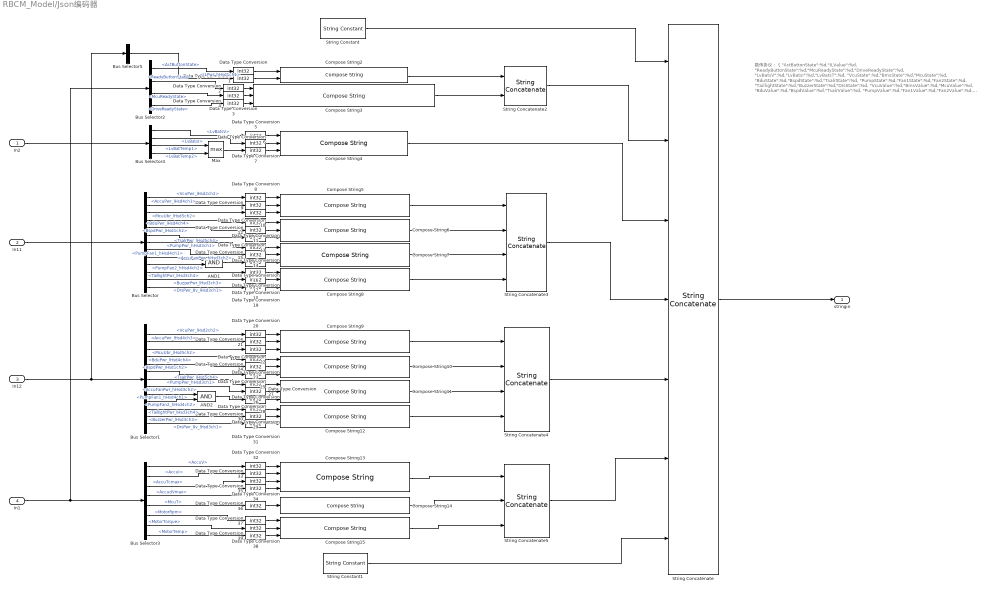
== system RBCM_Model/Json编码器 ==
  note: 数传协议：
      | {
      | "ActButtonState":%d,"ILValue":%d,
      | "ReadyButtonState":%d,"McuReadyState":%d,"DriveReadyState":%d,
      |
      | "LvBatsV":%d,"LvBatsI":%d,"LvBatsT":%d,
      |
      | "VcuState":%d,"BmsState":%d,"McuState":%d,
      | "BduState":%d,"BspdState":%d,"TsalrState":%d,
      | "PumpState":%d,"Fan1State":%d,"Fan2State":%d,
      | "TaillightState":%d,"BuzzerState":%d,"DrsState":%d,
      |
      | "VcuValue":%d,"BmsValue":%d,"McuValue":%d,
      | "BduValue":%d,"BspdValue":%d,"TsalrValue":%d,
      | "PumpValue":%d,"Fan1Value":%d,"Fan2Value":%d,
      | "TaillightValue":%d,"BuzzerValue":%d,"DrsValue":%d,
      |
      | "AccuV":%d,"AccuI":%d,"AccuTcmax":%d,"AccudVmax":%d,
      | "McuT":%d,
      | "MotorRpm":%d,"MotorTorque":%d,"MotorTemp":%d
      | }
  In2 : Inport  OutDataTypeStr=Bus: Bus_Vbats_Data
  In11 : Inport  Port=2  OutDataTypeStr=Bus: Bus_Hsd_Diagnose_Results
  In12 : Inport  Port=3  OutDataTypeStr=Bus: Bus_Hsd_Diagnose_Values
  In1 : Inport  Port=4  OutDataTypeStr=Bus: Bus_Vehicle_Data
  AND1 : Logic  IconShape=distinctive  AllPortsSameDT=off  OutDataTypeStr=boolean
  AND2 : Logic  IconShape=distinctive  AllPortsSameDT=off  OutDataTypeStr=boolean
  Bus Selector : BusSelector  OutputSignals=VcuPwr_lHsd2ch2,AccuPwr_lHsd4ch3,McuUbr_lHsd5ch2,BduPwr_lHsd4ch4,BspdPwr_lHsd1ch2,TsalrPwr_lHsd5ch4,PumpPwr_hHsd3ch1,AccuFanPwr_hHsd3ch2,PumpFan1_hHsd4ch1,PumpFan2_hHsd4ch2,TaillightPwr_lHsd3ch4,BuzzerPwr_lHsd3ch3,DrsPwr_8v_lHsd3ch1
  Bus Selector1 : BusSelector  OutputSignals=VcuPwr_lHsd2ch2,AccuPwr_lHsd4ch3,McuUbr_lHsd5ch2,BduPwr_lHsd4ch4,BspdPwr_lHsd1ch2,TsalrPwr_lHsd5ch4,PumpPwr_hHsd3ch1,AccuFanPwr_hHsd3ch2,PumpFan1_hHsd4ch1,PumpFan2_hHsd4ch2,TaillightPwr_lHsd3ch4,BuzzerPwr_lHsd3ch3,DrsPwr_8v_lHsd3ch1
  Bus Selector2 : BusSelector  OutputSignals=ActButtonState,ReadyButtonState,McuReadyState,DriveReadyState
  Bus Selector3 : BusSelector  OutputSignals=AccuV,AccuI,AccuTcmax,AccudVmax,McuT,MotorRpm,MotorTorque,MotorTemp
  Bus Selector4 : BusSelector  OutputSignals=LvBatsV,LvBatsI,LvBatTemp1,LvBatTemp2
  Bus Selector5 : BusSelector  OutputSignals=ILPwr_hHsd1ch1
  Compose String10 : ComposeString  Format="'\"BduValue\":%d,\"BspdValue\":%d,\"TsalrValue\":%d,'"
  Compose String11 : ComposeString  Format="'\"PumpValue\":%d,\"Fan1Value\":%d,\"Fan2Value\":%d,'"
  Compose String12 : ComposeString  Format="'\"TaillightValue\":%d,\"BuzzerValue\":%d,\"DrsValue\":%d,'"
  Compose String13 : ComposeString  Format="'\"AccuV\":%d,\"AccuI\":%d,\"AccuTcmax\":%d,\"AccudVmax\":%d,'"
  Compose String14 : ComposeString  Format="'\"McuT\":%d,'"
  Compose String15 : ComposeString  Format="'\"MotorRpm\":%d,\"MotorTorque\":%d,\"MotorTemp\":%d'"
  Compose String2 : ComposeString  Format="'\"ActButtonState\":%d,\"ILValue\":%d,'"
  Compose String3 : ComposeString  Format="'\"ReadyButtonState\":%d,\"McuReadyState\":%d,\"DriveReadyState\":%d,'"
  Compose String4 : ComposeString  Format="'\"LvBatsV\":%d,\"LvBatsI\":%d,\"LvBatsT\":%d,'"
  Compose String5 : ComposeString  Format="'\"VcuState\":%d,\"BmsState\":%d,\"McuState\":%d,'"
  Compose String6 : ComposeString  Format="'\"BduState\":%d,\"BspdState\":%d,\"TsalrState\":%d,'"
  Compose String7 : ComposeString  Format="'\"PumpValue\":%d,\"Fan1Value\":%d,\"Fan2Value\":%d,'"
  Compose String8 : ComposeString  Format="'\"TaillightValue\":%d,\"BuzzerValue\":%d,\"DrsValue\":%d,'"
  Compose String9 : ComposeString  Format="'\"VcuValue\":%d,\"BmsValue\":%d,\"McuValue\":%d,'"
  Data Type Conversion{,1..39} (40 alike) : DataTypeConversion  OutDataTypeStr=int32  SaturateOnIntegerOverflow=off  RndMeth=Floor
  Max : MinMax  Function=max  Inputs=2  OutDataTypeStr=uint16
  String Concatenate : StringConcatenate  Inputs=7
  String Concatenate2 : StringConcatenate
  String Concatenate3 : StringConcatenate  Inputs=4
  String Concatenate4 : StringConcatenate  Inputs=4
  String Concatenate5 : StringConcatenate  Inputs=3
  String Constant : StringConstant  String="\"{\""
  String Constant1 : StringConstant  String="\"}\""
  stringin : Outport
  wires:
  String Concatenate/1 -> stringin/1
  Compose String2/1 -> String Concatenate2/1
  Compose String3/1 -> String Concatenate2/2
  Compose String5/1 -> String Concatenate3/1
  Compose String6/1 -> String Concatenate3/2
  Compose String7/1 -> String Concatenate3/3
  Compose String8/1 -> String Concatenate3/4
  Compose String9/1 -> String Concatenate4/1
  Compose String10/1 -> String Concatenate4/2
  Compose String11/1 -> String Concatenate4/3
  Compose String12/1 -> String Concatenate4/4
  Compose String13/1 -> String Concatenate5/1
  Compose String14/1 -> String Concatenate5/2
  Compose String15/1 -> String Concatenate5/3
  String Constant/1 -> String Concatenate/1
  In11/1 -> Bus Selector/1
  In12/1 -> Bus Selector5/1, Bus Selector1/1
  In1/1 -> Bus Selector2/1, Bus Selector3/1
  String Concatenate2/1 -> String Concatenate/2
  Compose String4/1 -> String Concatenate/3
  String Concatenate3/1 -> String Concatenate/4
  String Concatenate4/1 -> String Concatenate/5
  String Concatenate5/1 -> String Concatenate/6
  String Constant1/1 -> String Concatenate/7
  Bus Selector2/1 -> Data Type Conversion/1  "<ActButtonState>"
  Bus Selector2/2 -> Data Type Conversion2/1  "<ReadyButtonState>"
  Bus Selector2/4 -> Data Type Conversion4/1  "<DriveReadyState>"
  Bus Selector2/3 -> Data Type Conversion3/1  "<McuReadyState>"
  In2/1 -> Bus Selector4/1
  Bus Selector4/1 -> Data Type Conversion5/1  "<LvBatsV>"
  Bus Selector4/2 -> Data Type Conversion7/1  "<LvBatsI>"
  Max/1 -> Data Type Conversion6/1
  Bus Selector4/3 -> Max/1  "<LvBatTemp1>"
  Bus Selector4/4 -> Max/2  "<LvBatTemp2>"
  Bus Selector5/1 -> Data Type Conversion1/1  "<ILPwr_hHsd1ch1>"
  Bus Selector/1 -> Data Type Conversion8/1  "<VcuPwr_lHsd2ch2>"
  Bus Selector/2 -> Data Type Conversion9/1  "<AccuPwr_lHsd4ch3>"
  Bus Selector/3 -> Data Type Conversion10/1  "<McuUbr_lHsd5ch2>"
  Bus Selector/4 -> Data Type Conversion11/1  "<BduPwr_lHsd4ch4>"
  Bus Selector/5 -> Data Type Conversion12/1  "<BspdPwr_lHsd1ch2>"
  Bus Selector/6 -> Data Type Conversion13/1  "<TsalrPwr_lHsd5ch4>"
  Bus Selector/7 -> Data Type Conversion14/1  "<PumpPwr_hHsd3ch1>"
  Bus Selector/8 -> Data Type Conversion15/1  "<AccuFanPwr_hHsd3ch2>"
  Bus Selector/9 -> AND1/1  "<PumpFan1_hHsd4ch1>"
  Bus Selector/10 -> AND1/2  "<PumpFan2_hHsd4ch2>"
  AND1/1 -> Data Type Conversion16/1
  Bus Selector/11 -> Data Type Conversion17/1  "<TaillightPwr_lHsd3ch4>"
  Bus Selector/12 -> Data Type Conversion18/1  "<BuzzerPwr_lHsd3ch3>"
  Bus Selector/13 -> Data Type Conversion19/1  "<DrsPwr_8v_lHsd3ch1>"
  Bus Selector1/1 -> Data Type Conversion20/1  "<VcuPwr_lHsd2ch2>"
  Bus Selector1/2 -> Data Type Conversion21/1  "<AccuPwr_lHsd4ch3>"
  Bus Selector1/3 -> Data Type Conversion22/1  "<McuUbr_lHsd5ch2>"
  Bus Selector1/4 -> Data Type Conversion23/1  "<BduPwr_lHsd4ch4>"
  Bus Selector1/5 -> Data Type Conversion24/1  "<BspdPwr_lHsd1ch2>"
  Bus Selector1/6 -> Data Type Conversion25/1  "<TsalrPwr_lHsd5ch4>"
  Bus Selector1/7 -> Data Type Conversion26/1  "<PumpPwr_hHsd3ch1>"
  Bus Selector1/8 -> Data Type Conversion27/1  "<AccuFanPwr_hHsd3ch2>"
  Bus Selector1/9 -> AND2/1  "<PumpFan1_hHsd4ch1>"
  Bus Selector1/10 -> AND2/2  "<PumpFan2_hHsd4ch2>"
  AND2/1 -> Data Type Conversion28/1
  Bus Selector1/11 -> Data Type Conversion29/1  "<TaillightPwr_lHsd3ch4>"
  Bus Selector1/12 -> Data Type Conversion30/1  "<BuzzerPwr_lHsd3ch3>"
  Bus Selector1/13 -> Data Type Conversion31/1  "<DrsPwr_8v_lHsd3ch1>"
  Bus Selector3/1 -> Data Type Conversion32/1  "<AccuV>"
  Bus Selector3/2 -> Data Type Conversion33/1  "<AccuI>"
  Bus Selector3/3 -> Data Type Conversion34/1  "<AccuTcmax>"
  Bus Selector3/4 -> Data Type Conversion35/1  "<AccudVmax>"
  Bus Selector3/5 -> Data Type Conversion36/1  "<McuT>"
  Bus Selector3/8 -> Data Type Conversion39/1  "<MotorTemp>"
  Bus Selector3/7 -> Data Type Conversion38/1  "<MotorTorque>"
  Bus Selector3/6 -> Data Type Conversion37/1  "<MotorRpm>"
  Data Type Conversion/1 -> Compose String2/1
  Data Type Conversion1/1 -> Compose String2/2
  Data Type Conversion2/1 -> Compose String3/1
  Data Type Conversion3/1 -> Compose String3/2
  Data Type Conversion4/1 -> Compose String3/3
  Data Type Conversion5/1 -> Compose String4/1
  Data Type Conversion6/1 -> Compose String4/3
  Data Type Conversion7/1 -> Compose String4/2
  Data Type Conversion8/1 -> Compose String5/1
  Data Type Conversion9/1 -> Compose String5/2
  Data Type Conversion10/1 -> Compose String5/3
  Data Type Conversion11/1 -> Compose String6/1
  Data Type Conversion12/1 -> Compose String6/2
  Data Type Conversion13/1 -> Compose String6/3
  Data Type Conversion14/1 -> Compose String7/1
  Data Type Conversion15/1 -> Compose String7/2
  Data Type Conversion16/1 -> Compose String7/3
  Data Type Conversion17/1 -> Compose String8/1
  Data Type Conversion18/1 -> Compose String8/2
  Data Type Conversion19/1 -> Compose String8/3
  Data Type Conversion20/1 -> Compose String9/1
  Data Type Conversion21/1 -> Compose String9/2
  Data Type Conversion22/1 -> Compose String9/3
  Data Type Conversion23/1 -> Compose String10/1
  Data Type Conversion24/1 -> Compose String10/2
  Data Type Conversion25/1 -> Compose String10/3
  Data Type Conversion26/1 -> Compose String11/1
  Data Type Conversion27/1 -> Compose String11/2
  Data Type Conversion28/1 -> Compose String11/3
  Data Type Conversion29/1 -> Compose String12/1
  Data Type Conversion30/1 -> Compose String12/2
  Data Type Conversion31/1 -> Compose String12/3
  Data Type Conversion32/1 -> Compose String13/1
  Data Type Conversion33/1 -> Compose String13/2
  Data Type Conversion34/1 -> Compose String13/3
  Data Type Conversion35/1 -> Compose String13/4
  Data Type Conversion36/1 -> Compose String14/1
  Data Type Conversion37/1 -> Compose String15/1
  Data Type Conversion38/1 -> Compose String15/2
  Data Type Conversion39/1 -> Compose String15/3
